simulink model "ss_co"  (R2017b)
settings: Solver=VariableStepAuto  StartTime=0.0  StopTime=10.0  RelTol=1e-3
values from neighbouring files (symbols this model uses):
  A = [0 657.92 0;0 0 1;0 -657.92 -40]    [ss_co.m]    (also in ss_co2.m)
  B = [0;0;1]    [ss_co.m]    (also in ss_co2.m)
settings Model: Creator=Luís Miranda  LastModifiedBy=Luís Miranda

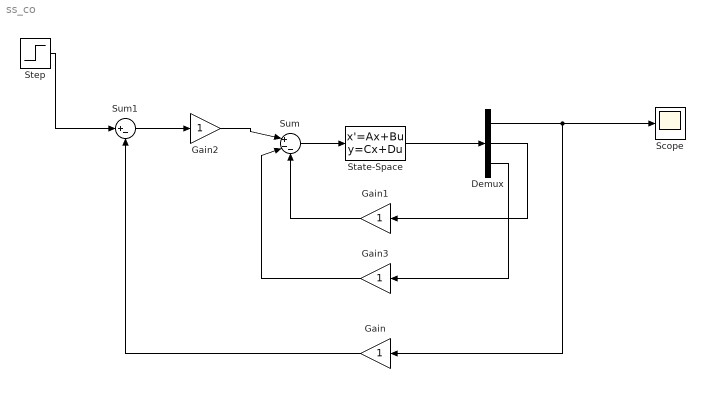
== system ss_co ==
  Demux : Demux  Outputs=3
  Gain{,1..3} (4 alike) : Gain
  Scope : Scope
  State-Space : StateSpace  A=A  B=B  C=eye(3)  D=[0; 0; 0]  InitialCondition=0
  Step : Step  SampleTime=0
  Sum : Sum  Inputs=|+--
  Sum1 : Sum  Inputs=|+-
  wires:
  Gain1/1 -> Sum/3
  Sum/1 -> State-Space/1
  Sum1/1 -> Gain2/1
  Step/1 -> Sum1/1
  Gain2/1 -> Sum/1
  Demux/3 -> Gain3/1
  Demux/1 -> Gain/1, Scope/1
  State-Space/1 -> Demux/1
  Demux/2 -> Gain1/1
  Gain3/1 -> Sum/2
  Gain/1 -> Sum1/2
